simulink model "Experiment1_model"  (R2022a)
settings: Solver=FixedStepAuto  StartTime=0.0  StopTime=20  RelTol=1e-3
libraries: slpidlib x32, slctrlblks x18
(part 4 of 5)

== system Experiment1_model/Robots Dynamics Decentralized1/Robot2 ==
  In1 : Inport
  Demux : Demux  Outputs=2
  Integrator : Integrator  InitialConditionSource=external  LimitOutput=on  UpperSaturationLimit=2  LowerSaturationLimit=-2
  Integrator1 : Integrator  InitialConditionSource=external
  initial conditions : Constant  Value=[0;0;-10;-10]  VectorParams1D=off
  p2 : Outport
  v2 : Outport  Port=2
  wires:
  initial conditions/1 -> Demux/1
  In1/1 -> Integrator/1  "u1"
  Demux/1 -> Integrator/2  "v0"
  Integrator/1 -> v2/1, Integrator1/1  "v"
  Demux/2 -> Integrator1/2  "p0"
  Integrator1/1 -> p2/1  "p"

== system Experiment1_model/Robots Dynamics Decentralized1/Robot3 ==
  In1 : Inport
  Demux : Demux  Outputs=2
  Integrator : Integrator  InitialConditionSource=external  LimitOutput=on  UpperSaturationLimit=2  LowerSaturationLimit=-2
  Integrator1 : Integrator  InitialConditionSource=external
  initial conditions : Constant  Value=[0;0;-10;10]  VectorParams1D=off
  p3 : Outport
  v3 : Outport  Port=2
  wires:
  initial conditions/1 -> Demux/1
  In1/1 -> Integrator/1  "u1"
  Demux/1 -> Integrator/2  "v0"
  Integrator/1 -> v3/1, Integrator1/1  "v"
  Demux/2 -> Integrator1/2  "p0"
  Integrator1/1 -> p3/1  "p"

== system Experiment1_model/Robots Dynamics Decentralized1/Robot4 ==
  In1 : Inport
  Demux : Demux  Outputs=2
  Integrator : Integrator  InitialConditionSource=external  LimitOutput=on  UpperSaturationLimit=2  LowerSaturationLimit=-2
  Integrator1 : Integrator  InitialConditionSource=external
  initial conditions : Constant  Value=[0;0;0;10]  VectorParams1D=off
  p4 : Outport
  v4 : Outport  Port=2
  wires:
  initial conditions/1 -> Demux/1
  In1/1 -> Integrator/1  "u1"
  Demux/1 -> Integrator/2  "v0"
  Integrator/1 -> v4/1, Integrator1/1  "v"
  Demux/2 -> Integrator1/2  "p0"
  Integrator1/1 -> p4/1  "p"

== system Experiment1_model/Robots Dynamics Decentralized1/Robot5 ==
  In1 : Inport
  Demux : Demux  Outputs=2
  Integrator : Integrator  InitialConditionSource=external  LimitOutput=on  UpperSaturationLimit=2  LowerSaturationLimit=-2
  Integrator1 : Integrator  InitialConditionSource=external
  initial conditions : Constant  Value=[0;0;-1;-10]  VectorParams1D=off
  p5 : Outport
  v5 : Outport  Port=2
  wires:
  initial conditions/1 -> Demux/1
  In1/1 -> Integrator/1  "u1"
  Demux/1 -> Integrator/2  "v0"
  Integrator/1 -> v5/1, Integrator1/1  "v"
  Demux/2 -> Integrator1/2  "p0"
  Integrator1/1 -> p5/1  "p"

== system Experiment1_model/Robots Dynamics Decentralized1/Robot6 ==
  In1 : Inport
  Demux : Demux  Outputs=2
  Integrator : Integrator  InitialConditionSource=external  LimitOutput=on  UpperSaturationLimit=2  LowerSaturationLimit=-2
  Integrator1 : Integrator  InitialConditionSource=external
  initial conditions : Constant  Value=[0;0;8;8]  VectorParams1D=off
  p6 : Outport
  v6 : Outport  Port=2
  wires:
  initial conditions/1 -> Demux/1
  In1/1 -> Integrator/1  "u1"
  Demux/1 -> Integrator/2  "v0"
  Integrator/1 -> v6/1, Integrator1/1  "v"
  Demux/2 -> Integrator1/2  "p0"
  Integrator1/1 -> p6/1  "p"

== system Experiment1_model/Robots Dynamics Decentralized1/Robot7 ==
  In1 : Inport
  Demux : Demux  Outputs=2
  Integrator : Integrator  InitialConditionSource=external  LimitOutput=on  UpperSaturationLimit=2  LowerSaturationLimit=-2
  Integrator1 : Integrator  InitialConditionSource=external
  initial conditions : Constant  Value=[0;0;10;-10]  VectorParams1D=off
  p7 : Outport
  v7 : Outport  Port=2
  wires:
  initial conditions/1 -> Demux/1
  In1/1 -> Integrator/1  "u1"
  Demux/1 -> Integrator/2  "v0"
  Integrator/1 -> v7/1, Integrator1/1  "v"
  Demux/2 -> Integrator1/2  "p0"
  Integrator1/1 -> p7/1  "p"

== system Experiment1_model/Robots Dynamics Decentralized1/Robot8 ==
  In1 : Inport
  Demux : Demux  Outputs=2
  Integrator : Integrator  InitialConditionSource=external  LimitOutput=on  UpperSaturationLimit=2  LowerSaturationLimit=-2
  Integrator1 : Integrator  InitialConditionSource=external
  initial conditions : Constant  Value=[0;0;12;-3]  VectorParams1D=off
  p8 : Outport
  v8 : Outport  Port=2
  wires:
  initial conditions/1 -> Demux/1
  In1/1 -> Integrator/1  "u1"
  Demux/1 -> Integrator/2  "v0"
  Integrator/1 -> v8/1, Integrator1/1  "v"
  Demux/2 -> Integrator1/2  "p0"
  Integrator1/1 -> p8/1  "p"

== system Experiment1_model/Robots Dynamics Decentralized1/Visualization ==
  p : Inport
  MATLAB Function : MATLAB Function  TreatAsAtomicUnit=on
  wires:
  p/1 -> MATLAB Function/1(p)

== system Experiment1_model/Robots Dynamics Decentralized1/Visualization1 ==
  p : Inport
  MATLAB Function : MATLAB Function  TreatAsAtomicUnit=on
  wires:
  p/1 -> MATLAB Function/1(p)

== system Experiment1_model/Safety CBF Enforcement Decentralized /CBF Robot1 ==
  states1 : Inport
  u01 : Inport  Port=2
  states : Inport  Port=3
  Barrier Certificate Enforcement : slctrlblks/Barrier Certificate Enforcement  nx=4  nu=2  nc=7  gamma=0.0025  beta=3  external_umax=on  external_umin=on  Ts=0.1  maxiter=200  tol=1e-6  output_exitflag=off
      settings: SourceProductBaseCode=SD
  Constant : Constant  Value=[zeros(2,2); eye(2)]
  Constant1 : Constant  Value=10*ones(2,1)
  Constant2 : Constant  Value=-10*ones(2,1)
  Gain : Gain  Gain=0.5
  Gain1 : Gain  Gain=[zeros(2), eye(2); zeros(2, 4)]  Multiplication=Matrix(K*u)
  dh : MATLAB Function  TreatAsAtomicUnit=on
  h : MATLAB Function  TreatAsAtomicUnit=on
  u_opt1 : Outport
  hx_1 : Outport  Port=2
  wires:
  Barrier Certificate Enforcement/1 -> u_opt1/1
  u01/1 -> Barrier Certificate Enforcement/1  "[2x1]"
  states/1 -> h/1(states), dh/1(states)
  Constant/1 -> Barrier Certificate Enforcement/3
  Constant1/1 -> Barrier Certificate Enforcement/6
  Constant2/1 -> Barrier Certificate Enforcement/7
  dh/1(qx1) -> Barrier Certificate Enforcement/5
  h/1(hx1) -> hx_1/1, Barrier Certificate Enforcement/4
  Gain/1 -> Barrier Certificate Enforcement/2
  states1/1 -> Gain1/1
  Gain1/1 -> Gain/1

== system Experiment1_model/Safety CBF Enforcement Decentralized /CBF Robot2 ==
  states2 : Inport
  u02 : Inport  Port=2
  states : Inport  Port=3
  Barrier Certificate Enforcement : slctrlblks/Barrier Certificate Enforcement  nx=4  nu=2  nc=7  gamma=0.0025  beta=3  external_umax=on  external_umin=on  Ts=0.1  maxiter=200  tol=1e-6  output_exitflag=off
      settings: SourceProductBaseCode=SD
  Constant : Constant  Value=[zeros(2,2); eye(2)]
  Constant1 : Constant  Value=10*ones(2,1)
  Constant2 : Constant  Value=-10*ones(2,1)
  Gain : Gain  Gain=0.5
  Gain1 : Gain  Gain=[zeros(2), eye(2); zeros(2, 4)]  Multiplication=Matrix(K*u)
  dh : MATLAB Function  TreatAsAtomicUnit=on
  h : MATLAB Function  TreatAsAtomicUnit=on
  u_opt2 : Outport
  wires:
  Barrier Certificate Enforcement/1 -> u_opt2/1
  u02/1 -> Barrier Certificate Enforcement/1  "[2x1]"
  states/1 -> h/1(states), dh/1(states)
  Constant/1 -> Barrier Certificate Enforcement/3
  Constant1/1 -> Barrier Certificate Enforcement/6
  Constant2/1 -> Barrier Certificate Enforcement/7
  dh/1(qx2) -> Barrier Certificate Enforcement/5
  h/1(hx2) -> Barrier Certificate Enforcement/4
  Gain/1 -> Barrier Certificate Enforcement/2
  Gain1/1 -> Gain/1
  states2/1 -> Gain1/1

== system Experiment1_model/Safety CBF Enforcement Decentralized /CBF Robot3 ==
  states3 : Inport
  u03 : Inport  Port=2
  states : Inport  Port=3
  Barrier Certificate Enforcement : slctrlblks/Barrier Certificate Enforcement  nx=4  nu=2  nc=7  gamma=0.0025  beta=3  external_umax=on  external_umin=on  Ts=0.1  maxiter=200  tol=1e-6  output_exitflag=off
      settings: SourceProductBaseCode=SD
  Constant : Constant  Value=[zeros(2,2); eye(2)]
  Constant1 : Constant  Value=10*ones(2,1)
  Constant2 : Constant  Value=-10*ones(2,1)
  Gain : Gain  Gain=0.5
  Gain1 : Gain  Gain=[zeros(2), eye(2); zeros(2, 4)]  Multiplication=Matrix(K*u)
  Scope : Scope
  dh : MATLAB Function  TreatAsAtomicUnit=on
  h : MATLAB Function  TreatAsAtomicUnit=on
  u_opt3 : Outport
  wires:
  Barrier Certificate Enforcement/1 -> u_opt3/1
  u03/1 -> Barrier Certificate Enforcement/1  "[2x1]"
  states/1 -> h/1(states), dh/1(states)
  Constant/1 -> Barrier Certificate Enforcement/3
  Constant1/1 -> Barrier Certificate Enforcement/6
  Constant2/1 -> Barrier Certificate Enforcement/7
  dh/1(qx3) -> Barrier Certificate Enforcement/5
  h/1(hx3) -> Scope/1, Barrier Certificate Enforcement/4
  Gain/1 -> Barrier Certificate Enforcement/2
  Gain1/1 -> Gain/1
  states3/1 -> Gain1/1

== system Experiment1_model/Safety CBF Enforcement Decentralized /CBF Robot4 ==
  states4 : Inport
  u04 : Inport  Port=2
  states : Inport  Port=3
  Barrier Certificate Enforcement : slctrlblks/Barrier Certificate Enforcement  nx=4  nu=2  nc=7  gamma=0.0025  beta=3  external_umax=on  external_umin=on  Ts=0.1  maxiter=200  tol=1e-6  output_exitflag=off
      settings: SourceProductBaseCode=SD
  Constant : Constant  Value=[zeros(2,2); eye(2)]
  Constant1 : Constant  Value=10*ones(2,1)
  Constant2 : Constant  Value=-10*ones(2,1)
  Gain : Gain  Gain=0.5
  Gain1 : Gain  Gain=[zeros(2), eye(2); zeros(2, 4)]  Multiplication=Matrix(K*u)
  dh : MATLAB Function  TreatAsAtomicUnit=on
  h : MATLAB Function  TreatAsAtomicUnit=on
  u_opt4 : Outport
  wires:
  Barrier Certificate Enforcement/1 -> u_opt4/1
  u04/1 -> Barrier Certificate Enforcement/1  "[2x1]"
  states/1 -> h/1(states), dh/1(states)
  Constant/1 -> Barrier Certificate Enforcement/3
  Constant1/1 -> Barrier Certificate Enforcement/6
  Constant2/1 -> Barrier Certificate Enforcement/7
  dh/1(qx4) -> Barrier Certificate Enforcement/5
  h/1(hx4) -> Barrier Certificate Enforcement/4
  Gain/1 -> Barrier Certificate Enforcement/2
  Gain1/1 -> Gain/1
  states4/1 -> Gain1/1

== system Experiment1_model/Safety CBF Enforcement Decentralized /CBF Robot5 ==
  states5 : Inport
  u05 : Inport  Port=2
  states : Inport  Port=3
  Barrier Certificate Enforcement : slctrlblks/Barrier Certificate Enforcement  nx=4  nu=2  nc=7  gamma=0.0025  beta=3  external_umax=on  external_umin=on  Ts=0.1  maxiter=200  tol=1e-6  output_exitflag=off
      settings: SourceProductBaseCode=SD
  Constant : Constant  Value=[zeros(2,2); eye(2)]
  Constant1 : Constant  Value=10*ones(2,1)
  Constant2 : Constant  Value=-10*ones(2,1)
  Gain : Gain  Gain=0.5
  Gain1 : Gain  Gain=[zeros(2), eye(2); zeros(2, 4)]  Multiplication=Matrix(K*u)
  dh : MATLAB Function  TreatAsAtomicUnit=on
  h : MATLAB Function  TreatAsAtomicUnit=on
  u_opt5 : Outport
  wires:
  Barrier Certificate Enforcement/1 -> u_opt5/1
  u05/1 -> Barrier Certificate Enforcement/1  "[2x1]"
  states/1 -> h/1(states), dh/1(states)
  Constant/1 -> Barrier Certificate Enforcement/3
  Constant1/1 -> Barrier Certificate Enforcement/6
  Constant2/1 -> Barrier Certificate Enforcement/7
  dh/1(qx5) -> Barrier Certificate Enforcement/5
  h/1(hx5) -> Barrier Certificate Enforcement/4
  Gain/1 -> Barrier Certificate Enforcement/2
  states5/1 -> Gain1/1
  Gain1/1 -> Gain/1

== system Experiment1_model/Safety CBF Enforcement Decentralized /CBF Robot6 ==
  states6 : Inport
  u06 : Inport  Port=2
  states : Inport  Port=3
  Barrier Certificate Enforcement : slctrlblks/Barrier Certificate Enforcement  nx=4  nu=2  nc=7  gamma=0.0025  beta=3  external_umax=on  external_umin=on  Ts=0.1  maxiter=200  tol=1e-6  output_exitflag=off
      settings: SourceProductBaseCode=SD
  Constant : Constant  Value=[zeros(2,2); eye(2)]
  Constant1 : Constant  Value=10*ones(2,1)
  Constant2 : Constant  Value=-10*ones(2,1)
  Gain : Gain  Gain=0.5
  Gain1 : Gain  Gain=[zeros(2), eye(2); zeros(2, 4)]  Multiplication=Matrix(K*u)
  dh : MATLAB Function  TreatAsAtomicUnit=on
  h : MATLAB Function  TreatAsAtomicUnit=on
  u_opt6 : Outport
  wires:
  Barrier Certificate Enforcement/1 -> u_opt6/1
  u06/1 -> Barrier Certificate Enforcement/1  "[2x1]"
  states/1 -> h/1(states), dh/1(states)
  Constant/1 -> Barrier Certificate Enforcement/3
  Constant1/1 -> Barrier Certificate Enforcement/6
  Constant2/1 -> Barrier Certificate Enforcement/7
  dh/1(qx6) -> Barrier Certificate Enforcement/5
  h/1(hx6) -> Barrier Certificate Enforcement/4
  Gain/1 -> Barrier Certificate Enforcement/2
  Gain1/1 -> Gain/1
  states6/1 -> Gain1/1

== system Experiment1_model/Safety CBF Enforcement Decentralized /CBF Robot7 ==
  states7 : Inport
  u07 : Inport  Port=2
  states : Inport  Port=3
  Barrier Certificate Enforcement : slctrlblks/Barrier Certificate Enforcement  nx=4  nu=2  nc=7  gamma=0.0025  beta=3  external_umax=on  external_umin=on  Ts=0.1  maxiter=200  tol=1e-6  output_exitflag=off
      settings: SourceProductBaseCode=SD
  Constant : Constant  Value=[zeros(2,2); eye(2)]
  Constant1 : Constant  Value=10*ones(2,1)
  Constant2 : Constant  Value=-10*ones(2,1)
  Gain : Gain  Gain=0.5
  Gain1 : Gain  Gain=[zeros(2), eye(2); zeros(2, 4)]  Multiplication=Matrix(K*u)
  dh : MATLAB Function  TreatAsAtomicUnit=on
  h : MATLAB Function  TreatAsAtomicUnit=on
  u_opt7 : Outport
  wires:
  Barrier Certificate Enforcement/1 -> u_opt7/1
  u07/1 -> Barrier Certificate Enforcement/1  "[2x1]"
  states/1 -> h/1(states), dh/1(states)
  Constant/1 -> Barrier Certificate Enforcement/3
  Constant1/1 -> Barrier Certificate Enforcement/6
  Constant2/1 -> Barrier Certificate Enforcement/7
  dh/1(qx7) -> Barrier Certificate Enforcement/5
  h/1(hx7) -> Barrier Certificate Enforcement/4
  Gain/1 -> Barrier Certificate Enforcement/2
  states7/1 -> Gain1/1
  Gain1/1 -> Gain/1

== system Experiment1_model/Safety CBF Enforcement Decentralized /CBF Robot8 ==
  states8 : Inport
  u08 : Inport  Port=2
  states : Inport  Port=3
  Barrier Certificate Enforcement : slctrlblks/Barrier Certificate Enforcement  nx=4  nu=2  nc=7  gamma=0.0025  beta=3  external_umax=on  external_umin=on  Ts=0.1  maxiter=200  tol=1e-6  output_exitflag=off
      settings: SourceProductBaseCode=SD
  Constant : Constant  Value=[zeros(2,2); eye(2)]
  Constant1 : Constant  Value=10*ones(2,1)
  Constant2 : Constant  Value=-10*ones(2,1)
  Gain : Gain  Gain=0.5
  Gain1 : Gain  Gain=[zeros(2), eye(2); zeros(2, 4)]  Multiplication=Matrix(K*u)
  dh : MATLAB Function  TreatAsAtomicUnit=on
  h : MATLAB Function  TreatAsAtomicUnit=on
  u_opt8 : Outport
  wires:
  Barrier Certificate Enforcement/1 -> u_opt8/1
  u08/1 -> Barrier Certificate Enforcement/1  "[2x1]"
  states/1 -> h/1(states), dh/1(states)
  Constant/1 -> Barrier Certificate Enforcement/3
  Constant1/1 -> Barrier Certificate Enforcement/6
  Constant2/1 -> Barrier Certificate Enforcement/7
  dh/1(qx8) -> Barrier Certificate Enforcement/5
  h/1(hx8) -> Barrier Certificate Enforcement/4
  Gain/1 -> Barrier Certificate Enforcement/2
  Gain1/1 -> Gain/1
  states8/1 -> Gain1/1

== system Experiment1_model/Safety CBF Enforcement Decentralized with Neighbours /CBF Robot1 ==
  states1 : Inport
  u01 : Inport  Port=2
  states : Inport  Port=3
  Barrier Certificate Enforcement : slctrlblks/Barrier Certificate Enforcement  nx=4  nu=2  nc=7  gamma=0.0025  beta=3  external_umax=on  external_umin=on  Ts=0.1  maxiter=200  tol=1e-6  output_exitflag=off
      settings: SourceProductBaseCode=SD
  Constant : Constant  Value=[zeros(2,2); eye(2)]
  Constant1 : Constant  Value=10*ones(2,1)
  Constant2 : Constant  Value=-10*ones(2,1)
  DeltaP : MATLAB Function  TreatAsAtomicUnit=on
  Gain : Gain  Gain=0.5
  Gain1 : Gain  Gain=[zeros(2), eye(2); zeros(2, 4)]  Multiplication=Matrix(K*u)
  Neighbourhood Radius : MATLAB Function  TreatAsAtomicUnit=on
  dh : MATLAB Function  TreatAsAtomicUnit=on
  h : MATLAB Function  TreatAsAtomicUnit=on
  u_opt1 : Outport
  Output : Outport  Port=2
  wires:
  Barrier Certificate Enforcement/1 -> u_opt1/1
  u01/1 -> Barrier Certificate Enforcement/1  "[2x1]"
  states/1 -> DeltaP/1(states), dh/1(states), h/1(states)
  Constant/1 -> Barrier Certificate Enforcement/3
  Constant1/1 -> Barrier Certificate Enforcement/6
  Constant2/1 -> Barrier Certificate Enforcement/7
  Gain/1 -> Barrier Certificate Enforcement/2
  states1/1 -> Gain1/1
  Gain1/1 -> Gain/1
  h/1(hx1) -> Neighbourhood Radius/1("hx1 ")
  dh/1(qx1) -> Neighbourhood Radius/2("qx1 ")
  DeltaP/1(deltaP1) -> Neighbourhood Radius/3(deltaP1)
  Neighbourhood Radius/1(hx1) -> Output/1, Barrier Certificate Enforcement/4
  Neighbourhood Radius/2(qx1) -> Barrier Certificate Enforcement/5

== system Experiment1_model/Safety CBF Enforcement Decentralized with Neighbours /CBF Robot2 ==
  states2 : Inport
  u02 : Inport  Port=2
  states : Inport  Port=3
  Barrier Certificate Enforcement : slctrlblks/Barrier Certificate Enforcement  nx=4  nu=2  nc=7  gamma=0.0025  beta=3  external_umax=on  external_umin=on  Ts=0.1  maxiter=200  tol=1e-6  output_exitflag=off
      settings: SourceProductBaseCode=SD
  Constant : Constant  Value=[zeros(2,2); eye(2)]
  Constant1 : Constant  Value=10*ones(2,1)
  Constant2 : Constant  Value=-10*ones(2,1)
  DeltaP : MATLAB Function  TreatAsAtomicUnit=on
  Gain : Gain  Gain=0.5
  Gain1 : Gain  Gain=[zeros(2), eye(2); zeros(2, 4)]  Multiplication=Matrix(K*u)
  Neighbourhood Radius : MATLAB Function  TreatAsAtomicUnit=on
  dh : MATLAB Function  TreatAsAtomicUnit=on
  h : MATLAB Function  TreatAsAtomicUnit=on
  u_opt2 : Outport
  wires:
  Barrier Certificate Enforcement/1 -> u_opt2/1
  u02/1 -> Barrier Certificate Enforcement/1  "[2x1]"
  states/1 -> dh/1(states), DeltaP/1(states), h/1(states)
  Constant/1 -> Barrier Certificate Enforcement/3
  Constant1/1 -> Barrier Certificate Enforcement/6
  Constant2/1 -> Barrier Certificate Enforcement/7
  Gain/1 -> Barrier Certificate Enforcement/2
  Gain1/1 -> Gain/1
  states2/1 -> Gain1/1
  Neighbourhood Radius/1(hx2) -> Barrier Certificate Enforcement/4
  Neighbourhood Radius/2(qx2) -> Barrier Certificate Enforcement/5
  DeltaP/1(deltaP2) -> Neighbourhood Radius/3(deltaP2)
  dh/1(qx2) -> Neighbourhood Radius/2("qx2 ")
  h/1(hx2) -> Neighbourhood Radius/1("hx2 ")

== system Experiment1_model/Safety CBF Enforcement Decentralized with Neighbours /CBF Robot3 ==
  states3 : Inport
  u03 : Inport  Port=2
  states : Inport  Port=3
  Barrier Certificate Enforcement : slctrlblks/Barrier Certificate Enforcement  nx=4  nu=2  nc=7  gamma=0.0025  beta=3  external_umax=on  external_umin=on  Ts=0.1  maxiter=200  tol=1e-6  output_exitflag=off
      settings: SourceProductBaseCode=SD
  Constant : Constant  Value=[zeros(2,2); eye(2)]
  Constant1 : Constant  Value=10*ones(2,1)
  Constant2 : Constant  Value=-10*ones(2,1)
  DeltaP : MATLAB Function  TreatAsAtomicUnit=on
  Gain : Gain  Gain=0.5
  Gain1 : Gain  Gain=[zeros(2), eye(2); zeros(2, 4)]  Multiplication=Matrix(K*u)
  Neighbourhood Radius : MATLAB Function  TreatAsAtomicUnit=on
  dh : MATLAB Function  TreatAsAtomicUnit=on
  h : MATLAB Function  TreatAsAtomicUnit=on
  u_opt3 : Outport
  wires:
  Barrier Certificate Enforcement/1 -> u_opt3/1
  u03/1 -> Barrier Certificate Enforcement/1  "[2x1]"
  states/1 -> dh/1(states), DeltaP/1(states), h/1(states)
  Constant/1 -> Barrier Certificate Enforcement/3
  Constant1/1 -> Barrier Certificate Enforcement/6
  Constant2/1 -> Barrier Certificate Enforcement/7
  Gain/1 -> Barrier Certificate Enforcement/2
  Gain1/1 -> Gain/1
  states3/1 -> Gain1/1
  Neighbourhood Radius/1(hx3) -> Barrier Certificate Enforcement/4
  Neighbourhood Radius/2(qx3) -> Barrier Certificate Enforcement/5
  DeltaP/1(deltaP3) -> Neighbourhood Radius/3(deltaP3)
  dh/1(qx3) -> Neighbourhood Radius/2("qx3 ")
  h/1(hx3) -> Neighbourhood Radius/1("hx3 ")

== system Experiment1_model/Safety CBF Enforcement Decentralized with Neighbours /CBF Robot4 ==
  states4 : Inport
  u04 : Inport  Port=2
  states : Inport  Port=3
  Barrier Certificate Enforcement : slctrlblks/Barrier Certificate Enforcement  nx=4  nu=2  nc=7  gamma=0.0025  beta=3  external_umax=on  external_umin=on  Ts=0.1  maxiter=200  tol=1e-6  output_exitflag=off
      settings: SourceProductBaseCode=SD
  Constant : Constant  Value=[zeros(2,2); eye(2)]
  Constant1 : Constant  Value=10*ones(2,1)
  Constant2 : Constant  Value=-10*ones(2,1)
  DeltaP : MATLAB Function  TreatAsAtomicUnit=on
  Gain : Gain  Gain=0.5
  Gain1 : Gain  Gain=[zeros(2), eye(2); zeros(2, 4)]  Multiplication=Matrix(K*u)
  Neighbourhood Radius : MATLAB Function  TreatAsAtomicUnit=on
  dh : MATLAB Function  TreatAsAtomicUnit=on
  h : MATLAB Function  TreatAsAtomicUnit=on
  u_opt4 : Outport
  wires:
  Barrier Certificate Enforcement/1 -> u_opt4/1
  u04/1 -> Barrier Certificate Enforcement/1  "[2x1]"
  states/1 -> DeltaP/1(states), dh/1(states), h/1(states)
  Constant/1 -> Barrier Certificate Enforcement/3
  Constant1/1 -> Barrier Certificate Enforcement/6
  Constant2/1 -> Barrier Certificate Enforcement/7
  Gain/1 -> Barrier Certificate Enforcement/2
  Gain1/1 -> Gain/1
  states4/1 -> Gain1/1
  Neighbourhood Radius/1(hx4) -> Barrier Certificate Enforcement/4
  Neighbourhood Radius/2(qx4) -> Barrier Certificate Enforcement/5
  dh/1(qx4) -> Neighbourhood Radius/2("qx4 ")
  DeltaP/1(deltaP4) -> Neighbourhood Radius/3(deltaP4)
  h/1(hx4) -> Neighbourhood Radius/1("hx4 ")

== system Experiment1_model/Safety CBF Enforcement Decentralized with Neighbours /CBF Robot5 ==
  states5 : Inport
  u05 : Inport  Port=2
  states : Inport  Port=3
  Barrier Certificate Enforcement : slctrlblks/Barrier Certificate Enforcement  nx=4  nu=2  nc=7  gamma=0.0025  beta=3  external_umax=on  external_umin=on  Ts=0.1  maxiter=200  tol=1e-6  output_exitflag=off
      settings: SourceProductBaseCode=SD
  Constant : Constant  Value=[zeros(2,2); eye(2)]
  Constant1 : Constant  Value=10*ones(2,1)
  Constant2 : Constant  Value=-10*ones(2,1)
  DeltaP : MATLAB Function  TreatAsAtomicUnit=on
  Gain : Gain  Gain=0.5
  Gain1 : Gain  Gain=[zeros(2), eye(2); zeros(2, 4)]  Multiplication=Matrix(K*u)
  Neighbourhood Radius : MATLAB Function  TreatAsAtomicUnit=on
  dh : MATLAB Function  TreatAsAtomicUnit=on
  h : MATLAB Function  TreatAsAtomicUnit=on
  u_opt5 : Outport
  wires:
  Barrier Certificate Enforcement/1 -> u_opt5/1
  u05/1 -> Barrier Certificate Enforcement/1  "[2x1]"
  states/1 -> DeltaP/1(states), dh/1(states), h/1(states)
  Constant/1 -> Barrier Certificate Enforcement/3
  Constant1/1 -> Barrier Certificate Enforcement/6
  Constant2/1 -> Barrier Certificate Enforcement/7
  Gain/1 -> Barrier Certificate Enforcement/2
  states5/1 -> Gain1/1
  Gain1/1 -> Gain/1
  Neighbourhood Radius/1(hx5) -> Barrier Certificate Enforcement/4
  Neighbourhood Radius/2(qx5) -> Barrier Certificate Enforcement/5
  DeltaP/1(deltaP5) -> Neighbourhood Radius/3(deltaP5)
  dh/1(qx5) -> Neighbourhood Radius/2("qx5 ")
  h/1(hx5) -> Neighbourhood Radius/1("hx5 ")

== system Experiment1_model/Safety CBF Enforcement Decentralized with Neighbours /CBF Robot6 ==
  states6 : Inport
  u06 : Inport  Port=2
  states : Inport  Port=3
  Barrier Certificate Enforcement : slctrlblks/Barrier Certificate Enforcement  nx=4  nu=2  nc=7  gamma=0.0025  beta=3  external_umax=on  external_umin=on  Ts=0.1  maxiter=200  tol=1e-6  output_exitflag=off
      settings: SourceProductBaseCode=SD
  Constant : Constant  Value=[zeros(2,2); eye(2)]
  Constant1 : Constant  Value=10*ones(2,1)
  Constant2 : Constant  Value=-10*ones(2,1)
  DeltaP : MATLAB Function  TreatAsAtomicUnit=on
  Gain : Gain  Gain=0.5
  Gain1 : Gain  Gain=[zeros(2), eye(2); zeros(2, 4)]  Multiplication=Matrix(K*u)
  Neighbourhood Radius : MATLAB Function  TreatAsAtomicUnit=on
  dh : MATLAB Function  TreatAsAtomicUnit=on
  h : MATLAB Function  TreatAsAtomicUnit=on
  u_opt6 : Outport
  wires:
  Barrier Certificate Enforcement/1 -> u_opt6/1
  u06/1 -> Barrier Certificate Enforcement/1  "[2x1]"
  states/1 -> DeltaP/1(states), dh/1(states), h/1(states)
  Constant/1 -> Barrier Certificate Enforcement/3
  Constant1/1 -> Barrier Certificate Enforcement/6
  Constant2/1 -> Barrier Certificate Enforcement/7
  Gain/1 -> Barrier Certificate Enforcement/2
  Gain1/1 -> Gain/1
  states6/1 -> Gain1/1
  Neighbourhood Radius/1(hx6) -> Barrier Certificate Enforcement/4
  Neighbourhood Radius/2(qx6) -> Barrier Certificate Enforcement/5
  DeltaP/1(deltaP6) -> Neighbourhood Radius/3(deltaP6)
  dh/1(qx6) -> Neighbourhood Radius/2("qx6 ")
  h/1(hx6) -> Neighbourhood Radius/1("hx6 ")

== system Experiment1_model/Safety CBF Enforcement Decentralized with Neighbours /CBF Robot7 ==
  states7 : Inport
  u07 : Inport  Port=2
  states : Inport  Port=3
  Barrier Certificate Enforcement : slctrlblks/Barrier Certificate Enforcement  nx=4  nu=2  nc=7  gamma=0.0025  beta=3  external_umax=on  external_umin=on  Ts=0.1  maxiter=200  tol=1e-6  output_exitflag=off
      settings: SourceProductBaseCode=SD
  Constant : Constant  Value=[zeros(2,2); eye(2)]
  Constant1 : Constant  Value=10*ones(2,1)
  Constant2 : Constant  Value=-10*ones(2,1)
  DeltaP : MATLAB Function  TreatAsAtomicUnit=on
  Gain : Gain  Gain=0.5
  Gain1 : Gain  Gain=[zeros(2), eye(2); zeros(2, 4)]  Multiplication=Matrix(K*u)
  Neighbourhood Radius : MATLAB Function  TreatAsAtomicUnit=on
  dh : MATLAB Function  TreatAsAtomicUnit=on
  h : MATLAB Function  TreatAsAtomicUnit=on
  u_opt7 : Outport
  wires:
  Barrier Certificate Enforcement/1 -> u_opt7/1
  u07/1 -> Barrier Certificate Enforcement/1  "[2x1]"
  states/1 -> DeltaP/1(states), dh/1(states), h/1(states)
  Constant/1 -> Barrier Certificate Enforcement/3
  Constant1/1 -> Barrier Certificate Enforcement/6
  Constant2/1 -> Barrier Certificate Enforcement/7
  Gain/1 -> Barrier Certificate Enforcement/2
  states7/1 -> Gain1/1
  Gain1/1 -> Gain/1
  Neighbourhood Radius/2(qx7) -> Barrier Certificate Enforcement/5
  Neighbourhood Radius/1(hx7) -> Barrier Certificate Enforcement/4
  DeltaP/1(deltaP7) -> Neighbourhood Radius/3(deltaP7)
  dh/1(qx7) -> Neighbourhood Radius/2("qx7 ")
  h/1(hx7) -> Neighbourhood Radius/1("hx7 ")

== system Experiment1_model/Safety CBF Enforcement Decentralized with Neighbours /CBF Robot8 ==
  states8 : Inport
  u08 : Inport  Port=2
  states : Inport  Port=3
  Barrier Certificate Enforcement : slctrlblks/Barrier Certificate Enforcement  nx=4  nu=2  nc=7  gamma=0.0025  beta=3  external_umax=on  external_umin=on  Ts=0.1  maxiter=200  tol=1e-6  output_exitflag=off
      settings: SourceProductBaseCode=SD
  Constant : Constant  Value=[zeros(2,2); eye(2)]
  Constant1 : Constant  Value=10*ones(2,1)
  Constant2 : Constant  Value=-10*ones(2,1)
  DeltaP : MATLAB Function  TreatAsAtomicUnit=on
  Gain : Gain  Gain=0.5
  Gain1 : Gain  Gain=[zeros(2), eye(2); zeros(2, 4)]  Multiplication=Matrix(K*u)
  Neighbourhood Radius : MATLAB Function  TreatAsAtomicUnit=on
  dh : MATLAB Function  TreatAsAtomicUnit=on
  h : MATLAB Function  TreatAsAtomicUnit=on
  u_opt8 : Outport
  wires:
  Barrier Certificate Enforcement/1 -> u_opt8/1
  u08/1 -> Barrier Certificate Enforcement/1  "[2x1]"
  states/1 -> DeltaP/1(states), dh/1(states), h/1(states)
  Constant/1 -> Barrier Certificate Enforcement/3
  Constant1/1 -> Barrier Certificate Enforcement/6
  Constant2/1 -> Barrier Certificate Enforcement/7
  Gain/1 -> Barrier Certificate Enforcement/2
  Gain1/1 -> Gain/1
  states8/1 -> Gain1/1
  Neighbourhood Radius/1(hx8) -> Barrier Certificate Enforcement/4
  Neighbourhood Radius/2(qx8) -> Barrier Certificate Enforcement/5
  DeltaP/1(deltaP8) -> Neighbourhood Radius/3(deltaP8)
  dh/1(qx8) -> Neighbourhood Radius/2("qx8 ")
  h/1(hx8) -> Neighbourhood Radius/1("hx8 ")

== matlab function Experiment1_model/Safety CBF Enforcement Decentralized /CBF Robot2/dh ==
  data: states input size=32; qx2 output size=[7 4]
function qx2 = fcn(states)
p1 = states(1:2);
p2 = states(3:4);
p3 = states(5:6);
p4 = states(7:8);
p5 = states(9:10);
p6 = states(11:12);
p7 = states(13:14);
p8 = states(15:16);

v1 = states(17:18);
v2 = states(19:20);
v3 = states(21:22);
v4 = states(23:24);
v5 = states(25:26);
v6 = states(27:28);
v7 = states(29:30);
v8 = states(31:32);

qx2 = CBF8Robots_dh2(states);

== matlab function Experiment1_model/Safety CBF Enforcement Decentralized /CBF Robot2/h ==
  data: states input size=32; hx2 output size=7
function hx2 = fcn(states)

p1 = states(1:2);
p2 = states(3:4);
p3 = states(5:6);
p4 = states(7:8);
p5 = states(9:10);
p6 = states(11:12);
p7 = states(13:14);
p8 = states(15:16);

v1 = states(17:18);
v2 = states(19:20);
v3 = states(21:22);
v4 = states(23:24);
v5 = states(25:26);
v6 = states(27:28);
v7 = states(29:30);
v8 = states(31:32);

hx2 = CBF8Robots_h2(states);

== matlab function Experiment1_model/Safety CBF Enforcement Decentralized /CBF Robot3/dh ==
  data: states input size=32; qx3 output size=[7 4]
function qx3 = fcn(states)
p1 = states(1:2);
p2 = states(3:4);
p3 = states(5:6);
p4 = states(7:8);
p5 = states(9:10);
p6 = states(11:12);
p7 = states(13:14);
p8 = states(15:16);

v1 = states(17:18);
v2 = states(19:20);
v3 = states(21:22);
v4 = states(23:24);
v5 = states(25:26);
v6 = states(27:28);
v7 = states(29:30);
v8 = states(31:32);

qx3 = CBF8Robots_dh3(states);

== matlab function Experiment1_model/Scopes/MATLAB Function ==
  data: hx1 input; hx1_12 output; hx2 input; hx2_12 output; hx3 input; hx4 input; hx3_12 output; hx4_12 output
function [hx1_12, hx2_12, hx3_12, hx4_12]  = fcn(hx1, hx2, hx3, hx4)

hx1_12 = hx1(1);
hx2_12 = hx2(1);
hx3_12 = hx3(1);
hx4_12 = hx4(1);

== matlab function Experiment1_model/Safety CBF Enforcement Decentralized /CBF Robot3/h ==
  data: states input size=32; hx3 output size=7
function hx3 = fcn(states)

p1 = states(1:2);
p2 = states(3:4);
p3 = states(5:6);
p4 = states(7:8);
p5 = states(9:10);
p6 = states(11:12);
p7 = states(13:14);
p8 = states(15:16);

v1 = states(17:18);
v2 = states(19:20);
v3 = states(21:22);
v4 = states(23:24);
v5 = states(25:26);
v6 = states(27:28);
v7 = states(29:30);
v8 = states(31:32);

hx3 = CBF8Robots_h3(states);

== matlab function Experiment1_model/Safety CBF Enforcement Decentralized /CBF Robot4/dh ==
  data: states input size=32; qx4 output size=[7 4]
function qx4 = fcn(states)
p1 = states(1:2);
p2 = states(3:4);
p3 = states(5:6);
p4 = states(7:8);
p5 = states(9:10);
p6 = states(11:12);
p7 = states(13:14);
p8 = states(15:16);

v1 = states(17:18);
v2 = states(19:20);
v3 = states(21:22);
v4 = states(23:24);
v5 = states(25:26);
v6 = states(27:28);
v7 = states(29:30);
v8 = states(31:32);

qx4 = CBF8Robots_dh4(states);

== matlab function Experiment1_model/Safety CBF Enforcement Centralized with Neighbours /MATLAB Function1 ==
  data: hx input; hx output; qx input; deltaP input; qx output
function [hx, qx] = fcn(hx, qx, deltaP)

E = 28;     % Maximum number of barriers
% Dn = 7;     % Fixed distance from neighbours

Ds = 0.5;   % Safe Distance


gamma = 0.3;

Dn = Ds + 1/(2*(10+10)) * ((2*(10+10)/gamma)^(1/2) + (2+2))^2;

for i=1:28
    if deltaP(i) >= Dn
        hx(i) = 0;
        qx(i,:) = 0;
    end
end

== matlab function Experiment1_model/Safety CBF Enforcement Centralized with Neighbours /dh ==
  data: states input size=32; qx output size=[28 32]
function qx = fcn(states)
p1 = states(1:2);
p2 = states(3:4);
p3 = states(5:6);
p4 = states(7:8);
p5 = states(9:10);
p6 = states(11:12);
p7 = states(13:14);
p8 = states(15:16);

v1 = states(17:18);
v2 = states(19:20);
v3 = states(21:22);
v4 = states(23:24);
v5 = states(25:26);
v6 = states(27:28);
v7 = states(29:30);
v8 = states(31:32);

qx = CBF8Robots_dh(states);

== matlab function Experiment1_model/Safety CBF Enforcement Centralized with Neighbours /h ==
  data: states input size=32; hx output size=28
function hx = fcn(states)

p1 = states(1:2);
p2 = states(3:4);
p3 = states(5:6);
p4 = states(7:8);
p5 = states(9:10);
p6 = states(11:12);
p7 = states(13:14);
p8 = states(15:16);

v1 = states(17:18);
v2 = states(19:20);
v3 = states(21:22);
v4 = states(23:24);
v5 = states(25:26);
v6 = states(27:28);
v7 = states(29:30);
v8 = states(31:32);

hx = CBF8Robots_h(states);

== matlab function Experiment1_model/Safety CBF Enforcement Decentralized /CBF Robot4/h ==
  data: states input size=32; hx4 output size=7
function hx4 = fcn(states)

p1 = states(1:2);
p2 = states(3:4);
p3 = states(5:6);
p4 = states(7:8);
p5 = states(9:10);
p6 = states(11:12);
p7 = states(13:14);
p8 = states(15:16);

v1 = states(17:18);
v2 = states(19:20);
v3 = states(21:22);
v4 = states(23:24);
v5 = states(25:26);
v6 = states(27:28);
v7 = states(29:30);
v8 = states(31:32);

hx4 = CBF8Robots_h4(states);

== matlab function Experiment1_model/Safety CBF Enforcement Decentralized /CBF Robot5/dh ==
  data: states input size=32; qx5 output size=[7 4]
function qx5 = fcn(states)
p1 = states(1:2);
p2 = states(3:4);
p3 = states(5:6);
p4 = states(7:8);
p5 = states(9:10);
p6 = states(11:12);
p7 = states(13:14);
p8 = states(15:16);

v1 = states(17:18);
v2 = states(19:20);
v3 = states(21:22);
v4 = states(23:24);
v5 = states(25:26);
v6 = states(27:28);
v7 = states(29:30);
v8 = states(31:32);

qx5 = CBF8Robots_dh5(states);

== matlab function Experiment1_model/Safety CBF Enforcement Decentralized /CBF Robot5/h ==
  data: states input size=32; hx5 output size=7
function hx5 = fcn(states)

p1 = states(1:2);
p2 = states(3:4);
p3 = states(5:6);
p4 = states(7:8);
p5 = states(9:10);
p6 = states(11:12);
p7 = states(13:14);
p8 = states(15:16);

v1 = states(17:18);
v2 = states(19:20);
v3 = states(21:22);
v4 = states(23:24);
v5 = states(25:26);
v6 = states(27:28);
v7 = states(29:30);
v8 = states(31:32);

hx5 = CBF8Robots_h5(states);

== matlab function Experiment1_model/Safety CBF Enforcement Decentralized /CBF Robot6/dh ==
  data: states input size=32; qx6 output size=[7 4]
function qx6 = fcn(states)
p1 = states(1:2);
p2 = states(3:4);
p3 = states(5:6);
p4 = states(7:8);
p5 = states(9:10);
p6 = states(11:12);
p7 = states(13:14);
p8 = states(15:16);

v1 = states(17:18);
v2 = states(19:20);
v3 = states(21:22);
v4 = states(23:24);
v5 = states(25:26);
v6 = states(27:28);
v7 = states(29:30);
v8 = states(31:32);

qx6 = CBF8Robots_dh6(states);

== matlab function Experiment1_model/Safety CBF Enforcement Decentralized /CBF Robot6/h ==
  data: states input size=32; hx6 output size=7
function hx6 = fcn(states)

p1 = states(1:2);
p2 = states(3:4);
p3 = states(5:6);
p4 = states(7:8);
p5 = states(9:10);
p6 = states(11:12);
p7 = states(13:14);
p8 = states(15:16);

v1 = states(17:18);
v2 = states(19:20);
v3 = states(21:22);
v4 = states(23:24);
v5 = states(25:26);
v6 = states(27:28);
v7 = states(29:30);
v8 = states(31:32);

hx6 = CBF8Robots_h6(states);

== matlab function Experiment1_model/Safety CBF Enforcement Decentralized /CBF Robot7/dh ==
  data: states input size=32; qx7 output size=[7 4]
function qx7 = fcn(states)
p1 = states(1:2);
p2 = states(3:4);
p3 = states(5:6);
p4 = states(7:8);
p5 = states(9:10);
p6 = states(11:12);
p7 = states(13:14);
p8 = states(15:16);

v1 = states(17:18);
v2 = states(19:20);
v3 = states(21:22);
v4 = states(23:24);
v5 = states(25:26);
v6 = states(27:28);
v7 = states(29:30);
v8 = states(31:32);

qx7 = CBF8Robots_dh7(states);

== matlab function Experiment1_model/Safety CBF Enforcement Decentralized /CBF Robot7/h ==
  data: states input size=32; hx7 output size=7
function hx7 = fcn(states)

p1 = states(1:2);
p2 = states(3:4);
p3 = states(5:6);
p4 = states(7:8);
p5 = states(9:10);
p6 = states(11:12);
p7 = states(13:14);
p8 = states(15:16);

v1 = states(17:18);
v2 = states(19:20);
v3 = states(21:22);
v4 = states(23:24);
v5 = states(25:26);
v6 = states(27:28);
v7 = states(29:30);
v8 = states(31:32);

hx7 = CBF8Robots_h7(states);

== matlab function Experiment1_model/Safety CBF Enforcement Decentralized /CBF Robot8/dh ==
  data: states input size=32; qx8 output size=[7 4]
function qx8 = fcn(states)
p1 = states(1:2);
p2 = states(3:4);
p3 = states(5:6);
p4 = states(7:8);
p5 = states(9:10);
p6 = states(11:12);
p7 = states(13:14);
p8 = states(15:16);

v1 = states(17:18);
v2 = states(19:20);
v3 = states(21:22);
v4 = states(23:24);
v5 = states(25:26);
v6 = states(27:28);
v7 = states(29:30);
v8 = states(31:32);

qx8 = CBF8Robots_dh8(states);

== matlab function Experiment1_model/Safety CBF Enforcement Decentralized /CBF Robot8/h ==
  data: states input size=32; hx8 output size=7
function hx8 = fcn(states)

p1 = states(1:2);
p2 = states(3:4);
p3 = states(5:6);
p4 = states(7:8);
p5 = states(9:10);
p6 = states(11:12);
p7 = states(13:14);
p8 = states(15:16);

v1 = states(17:18);
v2 = states(19:20);
v3 = states(21:22);
v4 = states(23:24);
v5 = states(25:26);
v6 = states(27:28);
v7 = states(29:30);
v8 = states(31:32);

hx8 = CBF8Robots_h8(states);

== matlab function Experiment1_model/Controller1 PID/Signal Routing ==
  data: states input; x_rob1 output; x_rob2 output; x_rob3 output; x_rob4 output; x_rob5 output; x_rob6 output; x_rob7 output; x_rob8 output
function [x_rob1, x_rob2, x_rob3, x_rob4, x_rob5, x_rob6, x_rob7, x_rob8] = fcn(states)


x_rob1 = [states(1); states(2); states(17); states(18)];
x_rob2 = [states(3); states(4); states(19); states(20)];
x_rob3 = [states(5); states(6); states(21); states(22)];
x_rob4 = [states(7); states(8); states(23); states(24)];
x_rob5 = [states(9); states(10); states(25); states(26)];
x_rob6 = [states(11); states(12); states(27); states(28)];
x_rob7 = [states(13); states(14); states(29); states(30)];
x_rob8 = [states(15); states(16); states(31); states(32)];

== matlab function Experiment1_model/Safety CBF Enforcement Decentralized with Neighbours /CBF Robot1/dh ==
  data: states input size=32; qx1 output size=[7 4]
function qx1 = fcn(states)
p1 = states(1:2);
p2 = states(3:4);
p3 = states(5:6);
p4 = states(7:8);
p5 = states(9:10);
p6 = states(11:12);
p7 = states(13:14);
p8 = states(15:16);

v1 = states(17:18);
v2 = states(19:20);
v3 = states(21:22);
v4 = states(23:24);
v5 = states(25:26);
v6 = states(27:28);
v7 = states(29:30);
v8 = states(31:32);

qx1 = CBF8Robots_dh1(states);

== matlab function Experiment1_model/Safety CBF Enforcement Decentralized with Neighbours /CBF Robot1/h ==
  data: states input size=32; hx1 output size=7
function hx1 = fcn(states)

p1 = states(1:2);
p2 = states(3:4);
p3 = states(5:6);
p4 = states(7:8);
p5 = states(9:10);
p6 = states(11:12);
p7 = states(13:14);
p8 = states(15:16);

v1 = states(17:18);
v2 = states(19:20);
v3 = states(21:22);
v4 = states(23:24);
v5 = states(25:26);
v6 = states(27:28);
v7 = states(29:30);
v8 = states(31:32);

hx1 = CBF8Robots_h1(states);

== matlab function Experiment1_model/Safety CBF Enforcement Decentralized with Neighbours /CBF Robot2/dh ==
  data: states input size=32; qx2 output size=[7 4]
function qx2 = fcn(states)
p1 = states(1:2);
p2 = states(3:4);
p3 = states(5:6);
p4 = states(7:8);
p5 = states(9:10);
p6 = states(11:12);
p7 = states(13:14);
p8 = states(15:16);

v1 = states(17:18);
v2 = states(19:20);
v3 = states(21:22);
v4 = states(23:24);
v5 = states(25:26);
v6 = states(27:28);
v7 = states(29:30);
v8 = states(31:32);

qx2 = CBF8Robots_dh2(states);

== matlab function Experiment1_model/Safety CBF Enforcement Decentralized with Neighbours /CBF Robot2/h ==
  data: states input size=32; hx2 output size=7
function hx2 = fcn(states)

p1 = states(1:2);
p2 = states(3:4);
p3 = states(5:6);
p4 = states(7:8);
p5 = states(9:10);
p6 = states(11:12);
p7 = states(13:14);
p8 = states(15:16);

v1 = states(17:18);
v2 = states(19:20);
v3 = states(21:22);
v4 = states(23:24);
v5 = states(25:26);
v6 = states(27:28);
v7 = states(29:30);
v8 = states(31:32);

hx2 = CBF8Robots_h2(states);

== matlab function Experiment1_model/Safety CBF Enforcement Decentralized with Neighbours /CBF Robot3/dh ==
  data: states input size=32; qx3 output size=[7 4]
function qx3 = fcn(states)
p1 = states(1:2);
p2 = states(3:4);
p3 = states(5:6);
p4 = states(7:8);
p5 = states(9:10);
p6 = states(11:12);
p7 = states(13:14);
p8 = states(15:16);

v1 = states(17:18);
v2 = states(19:20);
v3 = states(21:22);
v4 = states(23:24);
v5 = states(25:26);
v6 = states(27:28);
v7 = states(29:30);
v8 = states(31:32);

qx3 = CBF8Robots_dh3(states);

== matlab function Experiment1_model/Safety CBF Enforcement Decentralized with Neighbours /CBF Robot3/h ==
  data: states input size=32; hx3 output size=7
function hx3 = fcn(states)

p1 = states(1:2);
p2 = states(3:4);
p3 = states(5:6);
p4 = states(7:8);
p5 = states(9:10);
p6 = states(11:12);
p7 = states(13:14);
p8 = states(15:16);

v1 = states(17:18);
v2 = states(19:20);
v3 = states(21:22);
v4 = states(23:24);
v5 = states(25:26);
v6 = states(27:28);
v7 = states(29:30);
v8 = states(31:32);

hx3 = CBF8Robots_h3(states);

== matlab function Experiment1_model/Safety CBF Enforcement Decentralized with Neighbours /CBF Robot4/dh ==
  data: states input size=32; qx4 output size=[7 4]
function qx4 = fcn(states)
p1 = states(1:2);
p2 = states(3:4);
p3 = states(5:6);
p4 = states(7:8);
p5 = states(9:10);
p6 = states(11:12);
p7 = states(13:14);
p8 = states(15:16);

v1 = states(17:18);
v2 = states(19:20);
v3 = states(21:22);
v4 = states(23:24);
v5 = states(25:26);
v6 = states(27:28);
v7 = states(29:30);
v8 = states(31:32);

qx4 = CBF8Robots_dh4(states);

== matlab function Experiment1_model/Safety CBF Enforcement Decentralized with Neighbours /CBF Robot4/h ==
  data: states input size=32; hx4 output size=7
function hx4 = fcn(states)

p1 = states(1:2);
p2 = states(3:4);
p3 = states(5:6);
p4 = states(7:8);
p5 = states(9:10);
p6 = states(11:12);
p7 = states(13:14);
p8 = states(15:16);

v1 = states(17:18);
v2 = states(19:20);
v3 = states(21:22);
v4 = states(23:24);
v5 = states(25:26);
v6 = states(27:28);
v7 = states(29:30);
v8 = states(31:32);

hx4 = CBF8Robots_h4(states);

== matlab function Experiment1_model/Safety CBF Enforcement Decentralized with Neighbours /CBF Robot5/dh ==
  data: states input size=32; qx5 output size=[7 4]
function qx5 = fcn(states)
p1 = states(1:2);
p2 = states(3:4);
p3 = states(5:6);
p4 = states(7:8);
p5 = states(9:10);
p6 = states(11:12);
p7 = states(13:14);
p8 = states(15:16);

v1 = states(17:18);
v2 = states(19:20);
v3 = states(21:22);
v4 = states(23:24);
v5 = states(25:26);
v6 = states(27:28);
v7 = states(29:30);
v8 = states(31:32);

qx5 = CBF8Robots_dh5(states);

== matlab function Experiment1_model/Safety CBF Enforcement Decentralized with Neighbours /CBF Robot5/h ==
  data: states input size=32; hx5 output size=7
function hx5 = fcn(states)

p1 = states(1:2);
p2 = states(3:4);
p3 = states(5:6);
p4 = states(7:8);
p5 = states(9:10);
p6 = states(11:12);
p7 = states(13:14);
p8 = states(15:16);

v1 = states(17:18);
v2 = states(19:20);
v3 = states(21:22);
v4 = states(23:24);
v5 = states(25:26);
v6 = states(27:28);
v7 = states(29:30);
v8 = states(31:32);

hx5 = CBF8Robots_h5(states);

== matlab function Experiment1_model/Safety CBF Enforcement Decentralized with Neighbours /CBF Robot6/dh ==
  data: states input size=32; qx6 output size=[7 4]
function qx6 = fcn(states)
p1 = states(1:2);
p2 = states(3:4);
p3 = states(5:6);
p4 = states(7:8);
p5 = states(9:10);
p6 = states(11:12);
p7 = states(13:14);
p8 = states(15:16);

v1 = states(17:18);
v2 = states(19:20);
v3 = states(21:22);
v4 = states(23:24);
v5 = states(25:26);
v6 = states(27:28);
v7 = states(29:30);
v8 = states(31:32);

qx6 = CBF8Robots_dh6(states);

== matlab function Experiment1_model/Safety CBF Enforcement Decentralized with Neighbours /CBF Robot6/h ==
  data: states input size=32; hx6 output size=7
function hx6 = fcn(states)

p1 = states(1:2);
p2 = states(3:4);
p3 = states(5:6);
p4 = states(7:8);
p5 = states(9:10);
p6 = states(11:12);
p7 = states(13:14);
p8 = states(15:16);

v1 = states(17:18);
v2 = states(19:20);
v3 = states(21:22);
v4 = states(23:24);
v5 = states(25:26);
v6 = states(27:28);
v7 = states(29:30);
v8 = states(31:32);

hx6 = CBF8Robots_h6(states);

== matlab function Experiment1_model/Safety CBF Enforcement Decentralized with Neighbours /CBF Robot7/dh ==
  data: states input size=32; qx7 output size=[7 4]
function qx7 = fcn(states)
p1 = states(1:2);
p2 = states(3:4);
p3 = states(5:6);
p4 = states(7:8);
p5 = states(9:10);
p6 = states(11:12);
p7 = states(13:14);
p8 = states(15:16);

v1 = states(17:18);
v2 = states(19:20);
v3 = states(21:22);
v4 = states(23:24);
v5 = states(25:26);
v6 = states(27:28);
v7 = states(29:30);
v8 = states(31:32);

qx7 = CBF8Robots_dh7(states);

== matlab function Experiment1_model/Safety CBF Enforcement Decentralized with Neighbours /CBF Robot7/h ==
  data: states input size=32; hx7 output size=7
function hx7 = fcn(states)

p1 = states(1:2);
p2 = states(3:4);
p3 = states(5:6);
p4 = states(7:8);
p5 = states(9:10);
p6 = states(11:12);
p7 = states(13:14);
p8 = states(15:16);

v1 = states(17:18);
v2 = states(19:20);
v3 = states(21:22);
v4 = states(23:24);
v5 = states(25:26);
v6 = states(27:28);
v7 = states(29:30);
v8 = states(31:32);

hx7 = CBF8Robots_h7(states);

== matlab function Experiment1_model/Safety CBF Enforcement Decentralized with Neighbours /CBF Robot1/DeltaP ==
  data: states input; deltaP1 output
function deltaP1 = fcn(states)

p1 = states(1:2);
p2 = states(3:4);
p3 = states(5:6);
p4 = states(7:8);
p5 = states(9:10);
p6 = states(11:12);
p7 = states(13:14);
p8 = states(15:16);

v1 = states(17:18);
v2 = states(19:20);
v3 = states(21:22);
v4 = states(23:24);
v5 = states(25:26);
v6 = states(27:28);
v7 = states(29:30);
v8 = states(31:32);

deltaP1 = CBF8Robots_deltaP1(states);

== matlab function Experiment1_model/Safety CBF Enforcement Decentralized with Neighbours /CBF Robot1/Neighbourhood Radius ==
  data: hx1 input; hx1 output; qx1 input; deltaP1 input; qx1 output
function [hx1, qx1] = fcn(hx1, qx1, deltaP1)

E = 7;         % Maximum number of barriers
Ds = 0.6;      % Safe Distance
gamma = 0.3;   % Neighbour radius parameter 

Dn1 = Ds + 1/(2*(10+10)) * ((2*(10+10)/gamma)^(1/2) + (2+2))^2;

for i=1:E
    if deltaP1(i) >= Dn1
        hx1(i) = 0;
        qx1(i,:) = 0;
    end
end

== matlab function Experiment1_model/Safety CBF Enforcement Decentralized with Neighbours /CBF Robot2/DeltaP ==
  data: states input; deltaP2 output
function deltaP2 = fcn(states)

p1 = states(1:2);
p2 = states(3:4);
p3 = states(5:6);
p4 = states(7:8);
p5 = states(9:10);
p6 = states(11:12);
p7 = states(13:14);
p8 = states(15:16);

v1 = states(17:18);
v2 = states(19:20);
v3 = states(21:22);
v4 = states(23:24);
v5 = states(25:26);
v6 = states(27:28);
v7 = states(29:30);
v8 = states(31:32);

deltaP2 = CBF8Robots_deltaP2(states);

== matlab function Experiment1_model/Safety CBF Enforcement Decentralized with Neighbours /CBF Robot2/Neighbourhood Radius ==
  data: hx2 input; hx2 output; qx2 input; deltaP2 input; qx2 output
function [hx2, qx2] = fcn(hx2, qx2, deltaP2)

E = 7;         % Maximum number of barriers
Ds = 0.6;      % Safe Distance
gamma = 0.3;   % Neighbour radius parameter 

Dn2 = Ds + 1/(2*(10+10)) * ((2*(10+10)/gamma)^(1/2) + (2+2))^2;

for i=1:E
    if deltaP2(i) >= Dn2
        hx2(i) = 0;
        qx2(i,:) = 0;
    end
end

== matlab function Experiment1_model/Safety CBF Enforcement Decentralized with Neighbours /CBF Robot3/DeltaP ==
  data: states input; deltaP3 output
function deltaP3 = fcn(states)

p1 = states(1:2);
p2 = states(3:4);
p3 = states(5:6);
p4 = states(7:8);
p5 = states(9:10);
p6 = states(11:12);
p7 = states(13:14);
p8 = states(15:16);

v1 = states(17:18);
v2 = states(19:20);
v3 = states(21:22);
v4 = states(23:24);
v5 = states(25:26);
v6 = states(27:28);
v7 = states(29:30);
v8 = states(31:32);

deltaP3 = CBF8Robots_deltaP3(states);

== matlab function Experiment1_model/Robot Dynamics Centralized /Signal Reshaping ==
  data: p1 input; p output; v1 input; p2 input; v2 input; p3 input; v3 input; p4 input; v4 input; p5 input; v5 input; p6 input; v6 input; p7 input; v7 input; p8 input; v8 input; v output
function [p,v] = fcn(p1,v1,p2,v2,p3,v3,p4,v4,p5,v5,p6,v6,p7,v7,p8,v8)

p = [p1;p2;p3;p4;p5;p6;p7;p8;];
v = [v1;v2;v3;v4;v5;v6;v7;v8;];

== matlab function Experiment1_model/Safety CBF Enforcement Decentralized with Neighbours /CBF Robot3/Neighbourhood Radius ==
  data: hx3 input; hx3 output; qx3 input; deltaP3 input; qx3 output
function [hx3, qx3] = fcn(hx3, qx3, deltaP3)

E = 7;         % Maximum number of barriers
Ds = 0.6;      % Safe Distance
gamma = 0.3;   % Neighbour radius parameter 

Dn3 = Ds + 1/(2*(10+10)) * ((2*(10+10)/gamma)^(1/2) + (2+2))^2;

for i=1:E
    if deltaP3(i) >= Dn3
        hx3(i) = 0;
        qx3(i,:) = 0;
    end
end

== matlab function Experiment1_model/Safety CBF Enforcement Decentralized with Neighbours /CBF Robot4/DeltaP ==
  data: states input; deltaP4 output
function deltaP4 = fcn(states)

p1 = states(1:2);
p2 = states(3:4);
p3 = states(5:6);
p4 = states(7:8);
p5 = states(9:10);
p6 = states(11:12);
p7 = states(13:14);
p8 = states(15:16);

v1 = states(17:18);
v2 = states(19:20);
v3 = states(21:22);
v4 = states(23:24);
v5 = states(25:26);
v6 = states(27:28);
v7 = states(29:30);
v8 = states(31:32);

deltaP4 = CBF8Robots_deltaP4(states);

== matlab function Experiment1_model/Safety CBF Enforcement Decentralized with Neighbours /CBF Robot4/Neighbourhood Radius ==
  data: hx4 input; hx4 output; qx4 input; deltaP4 input; qx4 output
function [hx4, qx4] = fcn(hx4, qx4, deltaP4)

E = 7;         % Maximum number of barriers
Ds = 0.6;      % Safe Distance
gamma = 0.3;   % Neighbour radius parameter 

Dn4 = Ds + 1/(2*(10+10)) * ((2*(10+10)/gamma)^(1/2) + (2+2))^2;

for i=1:E
    if deltaP4(i) >= Dn4
        hx4(i) = 0;
        qx4(i,:) = 0;
    end
end

== matlab function Experiment1_model/Safety CBF Enforcement Decentralized with Neighbours /CBF Robot5/DeltaP ==
  data: states input; deltaP5 output
function deltaP5 = fcn(states)

p1 = states(1:2);
p2 = states(3:4);
p3 = states(5:6);
p4 = states(7:8);
p5 = states(9:10);
p6 = states(11:12);
p7 = states(13:14);
p8 = states(15:16);

v1 = states(17:18);
v2 = states(19:20);
v3 = states(21:22);
v4 = states(23:24);
v5 = states(25:26);
v6 = states(27:28);
v7 = states(29:30);
v8 = states(31:32);

deltaP5 = CBF8Robots_deltaP5(states);
